simulink model "bugfinder"  (R2017b)
settings: Solver=VariableStepAuto  StartTime=0.0  StopTime=10.0  RelTol=1e-3
libraries: simulink x1, CarLib x1
settings Model: Creator=Seb  LastModifiedBy=Seb

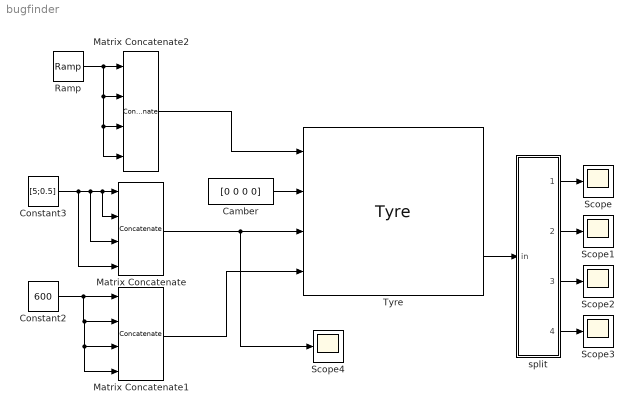
== system bugfinder ==
  Camber : Constant  Value=[0 0 0 0]  VectorParams1D=off
  Constant2 : Constant  Value=600
  Constant3 : Constant  Value=[5;0.5]
  Matrix Concatenate : Concatenate  NumInputs=4  Mode=Multidimensional array  ConcatenateDimension=2
  Matrix Concatenate1 : Concatenate  NumInputs=4  Mode=Multidimensional array  ConcatenateDimension=2
  Matrix Concatenate2 : Concatenate  NumInputs=4  Mode=Multidimensional array  ConcatenateDimension=2
  Ramp : simulink/Sources/Ramp  slope=4  start=0  X0=0
  Scope{,1..4} (5 alike) : Scope
  "Tyre " : CarLib/Tyre  tirfilename='Hoosier_43129_7inch_Round3.tir'
  split : MATLAB Function  TreatAsAtomicUnit=on
  wires:
  Matrix Concatenate/1 -> Scope4/1, "Tyre "/3
  Matrix Concatenate1/1 -> "Tyre "/4
  "Tyre "/2 -> split/1(in)
  Camber/1 -> "Tyre "/2
  Matrix Concatenate2/1 -> "Tyre "/1
  Ramp/1 -> Matrix Concatenate2/4, Matrix Concatenate2/3, Matrix Concatenate2/2, Matrix Concatenate2/1
  Constant3/1 -> Matrix Concatenate/4, Matrix Concatenate/3, Matrix Concatenate/2, Matrix Concatenate/1
  Constant2/1 -> Matrix Concatenate1/3, Matrix Concatenate1/4, Matrix Concatenate1/2, Matrix Concatenate1/1
  split/1(col1) -> Scope/1
  split/2(col2) -> Scope1/1
  split/3(col3) -> Scope2/1
  split/4(col4) -> Scope3/1

== matlab function bugfinder/split ==
  data: in input; col1 output; col2 output; col3 output; col4 output
function [col1,col2,col3,col4] = split(in)
    col1 = in(:,1);
    col2 = in(:,2);
    col3 = in(:,3);
    col4 = in(:,4);
end
